simulink model "untitled"  (R2023b)
settings: Solver=VariableStepAuto  StartTime=0.0  StopTime=10.0  RelTol=1e-3
libraries: sharedtransform x4, aerolibutil x1
settings Model: Creator=LENOVO  LastModifiedBy=LENOVO

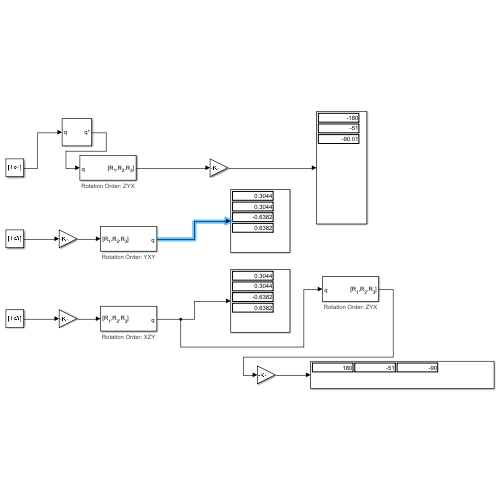
[thumbnail: Simulink's stored preview of the top-level diagram]
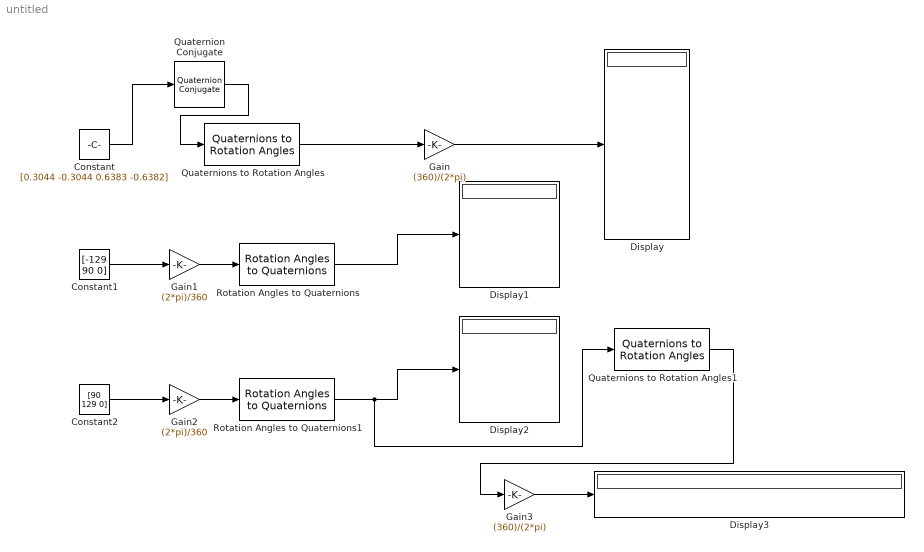
== system untitled ==
  Constant : Constant  Value=[0.3044 -0.3044 0.6383 -0.6382]
  Constant1 : Constant  Value=[-129 90 0]
  Constant2 : Constant  Value=[90 129 0]
  Display{,1..3} (4 alike) : Display
  Gain : Gain  Gain=(360)/(2*pi)
  Gain1 : Gain  Gain=(2*pi)/360
  Gain2 : Gain  Gain=(2*pi)/360
  Gain3 : Gain  Gain=(360)/(2*pi)
  Quaternion Conjugate : aerolibutil/Quaternion Conjugate
  Quaternions to Rotation Angles : sharedtransform/Quaternions to Rotation Angles  rotationOrder=ZYX  aMode=aMode
  Quaternions to Rotation Angles1 : sharedtransform/Quaternions to Rotation Angles  rotationOrder=ZYX  aMode=aMode
  Rotation Angles to Quaternions : sharedtransform/Rotation Angles to Quaternions  rotationOrder=YXY  aMode=aMode
  Rotation Angles to Quaternions1 : sharedtransform/Rotation Angles to Quaternions  rotationOrder=XZY  aMode=aMode
  wires:
  Constant/1 -> Quaternion Conjugate/1
  Quaternions to Rotation Angles/1 -> Gain/1
  Gain/1 -> Display/1
  Constant1/1 -> Gain1/1
  Gain1/1 -> Rotation Angles to Quaternions/1
  Rotation Angles to Quaternions/1 -> Display1/1
  Gain2/1 -> Rotation Angles to Quaternions1/1
  Rotation Angles to Quaternions1/1 -> Quaternions to Rotation Angles1/1, Display2/1
  Constant2/1 -> Gain2/1
  Quaternions to Rotation Angles1/1 -> Gain3/1
  Gain3/1 -> Display3/1
  Quaternion Conjugate/1 -> Quaternions to Rotation Angles/1
